simulink model "MMC_driven_PMSM_basic"  (R2025b)
settings: Solver=FixedStepDiscrete  StartTime=0.0  StopTime=7  FixedStep=Ts  RelTol=1e-3
values from neighbouring files (symbols this model uses):
  Goff = 1e-06    [initParams.mat]
  Ron = 1e-06    [initParams.mat]
  Ts = 5e-05    [initParams.mat]
  Vcell = 1000    [initParams.mat]
undefined symbols (not defined in the file or in its folder): DiscIntNeverNeededParam
libraries: ee_lib_for_power_systems x50, fl_lib x48, nesl_utility x3, eeTransforms x2, ee_lib x2, simulink x1
(part 2 of 2)

== system MMC_driven_PMSM_basic/MMC 8 Cell (Basic)/positive arm B/CELL 3 ==
  mod : Inport
  DC Voltage Source : fl_lib/Electrical/Electrical Sources/DC Voltage Source  v0=Vcell V
  Ideal Half-Bridge (Basic Diode) : ee_lib_for_power_systems/Power Converters/Ideal Half-Bridge (Basic Diode)  Ron=Ron  Goff=Goff  run_time=off
      settings: SourceProductName=Support Library for Power Systems
  + : PMIOPort  Side=Left
  - : PMIOPort  Port=2  Side=Left
  wires:
  mod/1 -> Ideal Half-Bridge (Basic Diode)/1
  connections:
  Ideal Half-Bridge (Basic Diode)/LConn1 -- +/RConn1
  Ideal Half-Bridge (Basic Diode)/RConn1 -- DC Voltage Source/LConn1
  Ideal Half-Bridge (Basic Diode)/RConn2 -- DC Voltage Source/RConn1 -- -/RConn1

== system MMC_driven_PMSM_basic/MMC 8 Cell (Basic)/positive arm B/CELL 4 ==
  mod : Inport
  DC Voltage Source : fl_lib/Electrical/Electrical Sources/DC Voltage Source  v0=Vcell V
  Ideal Half-Bridge (Basic Diode) : ee_lib_for_power_systems/Power Converters/Ideal Half-Bridge (Basic Diode)  Ron=Ron  Goff=Goff  run_time=off
      settings: SourceProductName=Support Library for Power Systems
  + : PMIOPort  Side=Left
  - : PMIOPort  Port=2  Side=Left
  wires:
  mod/1 -> Ideal Half-Bridge (Basic Diode)/1
  connections:
  -/RConn1 -- DC Voltage Source/RConn1 -- Ideal Half-Bridge (Basic Diode)/RConn2
  Ideal Half-Bridge (Basic Diode)/RConn1 -- DC Voltage Source/LConn1
  Ideal Half-Bridge (Basic Diode)/LConn1 -- +/RConn1

== system MMC_driven_PMSM_basic/MMC 8 Cell (Basic)/positive arm B/CELL 5 ==
  mod : Inport
  DC Voltage Source : fl_lib/Electrical/Electrical Sources/DC Voltage Source  v0=Vcell V
  Ideal Half-Bridge (Basic Diode) : ee_lib_for_power_systems/Power Converters/Ideal Half-Bridge (Basic Diode)  Ron=Ron  Goff=Goff  run_time=off
      settings: SourceProductName=Support Library for Power Systems
  + : PMIOPort  Side=Left
  - : PMIOPort  Port=2  Side=Left
  wires:
  mod/1 -> Ideal Half-Bridge (Basic Diode)/1
  connections:
  Ideal Half-Bridge (Basic Diode)/LConn1 -- +/RConn1
  Ideal Half-Bridge (Basic Diode)/RConn1 -- DC Voltage Source/LConn1
  Ideal Half-Bridge (Basic Diode)/RConn2 -- DC Voltage Source/RConn1 -- -/RConn1

== system MMC_driven_PMSM_basic/MMC 8 Cell (Basic)/positive arm B/CELL 6 ==
  mod : Inport
  DC Voltage Source : fl_lib/Electrical/Electrical Sources/DC Voltage Source  v0=Vcell V
  Ideal Half-Bridge (Basic Diode) : ee_lib_for_power_systems/Power Converters/Ideal Half-Bridge (Basic Diode)  Ron=Ron  Goff=Goff  run_time=off
      settings: SourceProductName=Support Library for Power Systems
  + : PMIOPort  Side=Left
  - : PMIOPort  Port=2  Side=Left
  wires:
  mod/1 -> Ideal Half-Bridge (Basic Diode)/1
  connections:
  -/RConn1 -- DC Voltage Source/RConn1 -- Ideal Half-Bridge (Basic Diode)/RConn2
  Ideal Half-Bridge (Basic Diode)/RConn1 -- DC Voltage Source/LConn1
  Ideal Half-Bridge (Basic Diode)/LConn1 -- +/RConn1

== system MMC_driven_PMSM_basic/MMC 8 Cell (Basic)/positive arm B/CELL 7 ==
  mod : Inport
  DC Voltage Source : fl_lib/Electrical/Electrical Sources/DC Voltage Source  v0=Vcell V
  Ideal Half-Bridge (Basic Diode) : ee_lib_for_power_systems/Power Converters/Ideal Half-Bridge (Basic Diode)  Ron=Ron  Goff=Goff  run_time=off
      settings: SourceProductName=Support Library for Power Systems
  + : PMIOPort  Side=Left
  - : PMIOPort  Port=2  Side=Left
  wires:
  mod/1 -> Ideal Half-Bridge (Basic Diode)/1
  connections:
  Ideal Half-Bridge (Basic Diode)/LConn1 -- +/RConn1
  Ideal Half-Bridge (Basic Diode)/RConn1 -- DC Voltage Source/LConn1
  Ideal Half-Bridge (Basic Diode)/RConn2 -- DC Voltage Source/RConn1 -- -/RConn1

== system MMC_driven_PMSM_basic/MMC 8 Cell (Basic)/positive arm B/CELL 8 ==
  mod : Inport
  DC Voltage Source : fl_lib/Electrical/Electrical Sources/DC Voltage Source  v0=Vcell V
  Ideal Half-Bridge (Basic Diode) : ee_lib_for_power_systems/Power Converters/Ideal Half-Bridge (Basic Diode)  Ron=Ron  Goff=Goff  run_time=off
      settings: SourceProductName=Support Library for Power Systems
  + : PMIOPort  Side=Left
  - : PMIOPort  Port=2  Side=Left
  wires:
  mod/1 -> Ideal Half-Bridge (Basic Diode)/1
  connections:
  -/RConn1 -- DC Voltage Source/RConn1 -- Ideal Half-Bridge (Basic Diode)/RConn2
  Ideal Half-Bridge (Basic Diode)/RConn1 -- DC Voltage Source/LConn1
  Ideal Half-Bridge (Basic Diode)/LConn1 -- +/RConn1

== system MMC_driven_PMSM_basic/MMC 8 Cell (Basic)/positive arm C/CELL 1 ==
  mod : Inport
  DC Voltage Source : fl_lib/Electrical/Electrical Sources/DC Voltage Source  v0=Vcell V
  Ideal Half-Bridge (Basic Diode) : ee_lib_for_power_systems/Power Converters/Ideal Half-Bridge (Basic Diode)  Ron=Ron  Goff=Goff  run_time=off
      settings: SourceProductName=Support Library for Power Systems
  + : PMIOPort  Side=Left
  - : PMIOPort  Port=2  Side=Left
  wires:
  mod/1 -> Ideal Half-Bridge (Basic Diode)/1
  connections:
  -/RConn1 -- DC Voltage Source/RConn1 -- Ideal Half-Bridge (Basic Diode)/RConn2
  Ideal Half-Bridge (Basic Diode)/RConn1 -- DC Voltage Source/LConn1
  Ideal Half-Bridge (Basic Diode)/LConn1 -- +/RConn1

== system MMC_driven_PMSM_basic/MMC 8 Cell (Basic)/positive arm C/CELL 2 ==
  mod : Inport
  DC Voltage Source : fl_lib/Electrical/Electrical Sources/DC Voltage Source  v0=Vcell V
  Ideal Half-Bridge (Basic Diode) : ee_lib_for_power_systems/Power Converters/Ideal Half-Bridge (Basic Diode)  Ron=Ron  Goff=Goff  run_time=off
      settings: SourceProductName=Support Library for Power Systems
  + : PMIOPort  Side=Left
  - : PMIOPort  Port=2  Side=Left
  wires:
  mod/1 -> Ideal Half-Bridge (Basic Diode)/1
  connections:
  Ideal Half-Bridge (Basic Diode)/LConn1 -- +/RConn1
  Ideal Half-Bridge (Basic Diode)/RConn1 -- DC Voltage Source/LConn1
  Ideal Half-Bridge (Basic Diode)/RConn2 -- DC Voltage Source/RConn1 -- -/RConn1

== system MMC_driven_PMSM_basic/MMC 8 Cell (Basic)/positive arm C/CELL 3 ==
  mod : Inport
  DC Voltage Source : fl_lib/Electrical/Electrical Sources/DC Voltage Source  v0=Vcell V
  Ideal Half-Bridge (Basic Diode) : ee_lib_for_power_systems/Power Converters/Ideal Half-Bridge (Basic Diode)  Ron=Ron  Goff=Goff  run_time=off
      settings: SourceProductName=Support Library for Power Systems
  + : PMIOPort  Side=Left
  - : PMIOPort  Port=2  Side=Left
  wires:
  mod/1 -> Ideal Half-Bridge (Basic Diode)/1
  connections:
  -/RConn1 -- DC Voltage Source/RConn1 -- Ideal Half-Bridge (Basic Diode)/RConn2
  Ideal Half-Bridge (Basic Diode)/RConn1 -- DC Voltage Source/LConn1
  Ideal Half-Bridge (Basic Diode)/LConn1 -- +/RConn1

== system MMC_driven_PMSM_basic/MMC 8 Cell (Basic)/positive arm C/CELL 4 ==
  mod : Inport
  DC Voltage Source : fl_lib/Electrical/Electrical Sources/DC Voltage Source  v0=Vcell V
  Ideal Half-Bridge (Basic Diode) : ee_lib_for_power_systems/Power Converters/Ideal Half-Bridge (Basic Diode)  Ron=Ron  Goff=Goff  run_time=off
      settings: SourceProductName=Support Library for Power Systems
  + : PMIOPort  Side=Left
  - : PMIOPort  Port=2  Side=Left
  wires:
  mod/1 -> Ideal Half-Bridge (Basic Diode)/1
  connections:
  Ideal Half-Bridge (Basic Diode)/LConn1 -- +/RConn1
  Ideal Half-Bridge (Basic Diode)/RConn1 -- DC Voltage Source/LConn1
  Ideal Half-Bridge (Basic Diode)/RConn2 -- DC Voltage Source/RConn1 -- -/RConn1

== system MMC_driven_PMSM_basic/MMC 8 Cell (Basic)/positive arm C/CELL 5 ==
  mod : Inport
  DC Voltage Source : fl_lib/Electrical/Electrical Sources/DC Voltage Source  v0=Vcell V
  Ideal Half-Bridge (Basic Diode) : ee_lib_for_power_systems/Power Converters/Ideal Half-Bridge (Basic Diode)  Ron=Ron  Goff=Goff  run_time=off
      settings: SourceProductName=Support Library for Power Systems
  + : PMIOPort  Side=Left
  - : PMIOPort  Port=2  Side=Left
  wires:
  mod/1 -> Ideal Half-Bridge (Basic Diode)/1
  connections:
  -/RConn1 -- DC Voltage Source/RConn1 -- Ideal Half-Bridge (Basic Diode)/RConn2
  Ideal Half-Bridge (Basic Diode)/RConn1 -- DC Voltage Source/LConn1
  Ideal Half-Bridge (Basic Diode)/LConn1 -- +/RConn1

== system MMC_driven_PMSM_basic/MMC 8 Cell (Basic)/positive arm C/CELL 6 ==
  mod : Inport
  DC Voltage Source : fl_lib/Electrical/Electrical Sources/DC Voltage Source  v0=Vcell V
  Ideal Half-Bridge (Basic Diode) : ee_lib_for_power_systems/Power Converters/Ideal Half-Bridge (Basic Diode)  Ron=Ron  Goff=Goff  run_time=off
      settings: SourceProductName=Support Library for Power Systems
  + : PMIOPort  Side=Left
  - : PMIOPort  Port=2  Side=Left
  wires:
  mod/1 -> Ideal Half-Bridge (Basic Diode)/1
  connections:
  Ideal Half-Bridge (Basic Diode)/LConn1 -- +/RConn1
  Ideal Half-Bridge (Basic Diode)/RConn1 -- DC Voltage Source/LConn1
  Ideal Half-Bridge (Basic Diode)/RConn2 -- DC Voltage Source/RConn1 -- -/RConn1

== system MMC_driven_PMSM_basic/MMC 8 Cell (Basic)/positive arm C/CELL 7 ==
  mod : Inport
  DC Voltage Source : fl_lib/Electrical/Electrical Sources/DC Voltage Source  v0=Vcell V
  Ideal Half-Bridge (Basic Diode) : ee_lib_for_power_systems/Power Converters/Ideal Half-Bridge (Basic Diode)  Ron=Ron  Goff=Goff  run_time=off
      settings: SourceProductName=Support Library for Power Systems
  + : PMIOPort  Side=Left
  - : PMIOPort  Port=2  Side=Left
  wires:
  mod/1 -> Ideal Half-Bridge (Basic Diode)/1
  connections:
  -/RConn1 -- DC Voltage Source/RConn1 -- Ideal Half-Bridge (Basic Diode)/RConn2
  Ideal Half-Bridge (Basic Diode)/RConn1 -- DC Voltage Source/LConn1
  Ideal Half-Bridge (Basic Diode)/LConn1 -- +/RConn1

== system MMC_driven_PMSM_basic/MMC 8 Cell (Basic)/positive arm C/CELL 8 ==
  mod : Inport
  DC Voltage Source : fl_lib/Electrical/Electrical Sources/DC Voltage Source  v0=Vcell V
  Ideal Half-Bridge (Basic Diode) : ee_lib_for_power_systems/Power Converters/Ideal Half-Bridge (Basic Diode)  Ron=Ron  Goff=Goff  run_time=off
      settings: SourceProductName=Support Library for Power Systems
  + : PMIOPort  Side=Left
  - : PMIOPort  Port=2  Side=Left
  wires:
  mod/1 -> Ideal Half-Bridge (Basic Diode)/1
  connections:
  Ideal Half-Bridge (Basic Diode)/LConn1 -- +/RConn1
  Ideal Half-Bridge (Basic Diode)/RConn1 -- DC Voltage Source/LConn1
  Ideal Half-Bridge (Basic Diode)/RConn2 -- DC Voltage Source/RConn1 -- -/RConn1
